simulink library "inp"  (R2021b)
settings: Solver=VariableStepAuto  StartTime=0.0  StopTime=10.0  RelTol=1e-3
undefined symbols (not defined in the file): C_TASK_5MS_S, FALSE, KINP_AcoreReadyToSlp_flg_ovrdflg, KINP_AcoreReadyToSlp_flg_ovrdval, KINP_AllowMovThd_OTA_enum_ovrdflg, KINP_AllowMovThd_OTA_enum_ovrdval, KINP_APSAngleTarget_Deg_ovrdflg, KINP_APSAngleTarget_Deg_ovrdval, KINP_APSDecReq_mps2_ovrdflg, KINP_APSDecReq_mps2_ovrdval, KINP_APSDecReqA_flg_ovrdflg, KINP_APSDecReqA_flg_ovrdval, KINP_APSDFLL_cm_ovrdflg, KINP_APSDFLL_cm_ovrdval, KINP_APSDFLR_cm_ovrdflg, KINP_APSDFLR_cm_ovrdval, KINP_APSDRLL_cm_ovrdflg, KINP_APSDRLL_cm_ovrdval, KINP_APSDRLR_cm_ovrdflg, KINP_APSDRLR_cm_ovrdval, KINP_APSExitCondition_enum_ovrdflg, KINP_APSExitCondition_enum_ovrdval, KINP_APSHWVer_enum_ovrdflg, KINP_APSHWVer_enum_ovrdval, KINP_APSProgressPCT_pct_ovrdflg, KINP_APSProgressPCT_pct_ovrdval, KINP_APSPwrReq_enum_ovrdflg, KINP_APSPwrReq_enum_ovrdval, KINP_APSReq_enum_ovrdflg, KINP_APSReq_enum_ovrdval, KINP_APSRQDisplay_enum_ovrdflg, KINP_APSRQDisplay_enum_ovrdval, KINP_APSRqEPASCtrl_flg_ovrdflg, KINP_APSRqEPASCtrl_flg_ovrdval, KINP_APSShiftPosnReq_enum_ovrdval, KINP_APSShiftPosnReq_enum_ovrflg, KINP_APSSpeedCMD_kph_ovrdval, KINP_APSSpeedCMD_kph_ovrflg, KINP_APSStaSystem_enum_ovrdflg, KINP_APSStaSystem_enum_ovrdval, KINP_APSSWVer_enum_ovrdflg, KINP_APSSWVer_enum_ovrdval, KINP_APSVMCReqA_flg_ovrdval, KINP_APSVMCReqA_flg_ovrflg, KINP_APSVRqEPASCtrl_flg_ovrdflg, KINP_APSVRqEPASCtrl_flg_ovrdval, KINP_AuxBattVolmV_mV_ovrdflg, KINP_AuxBattVolmV_mV_ovrdval, KINP_BTConnectSta_enum_ovrdflg, KINP_BTConnectSta_enum_ovrdval, KINP_CAASSta_enum_ovrdflg, KINP_CAASSta_enum_ovrdval, KINP_CAASVMCReqA_flg_ovrdval, KINP_CAASVMCReqA_flg_ovrflg, KINP_CAN1BusOff_flg_ovrdflg, KINP_CAN1BusOff_flg_ovrdval, KINP_CAN2BusOff_flg_ovrdflg, KINP_CAN2BusOff_flg_ovrdval, KINP_CAN3BusOff_flg_ovrdflg, KINP_CAN3BusOff_flg_ovrdval ... (+158)
libraries: FVT_lib x184, hcu_lib x1
(part 8 of 8)

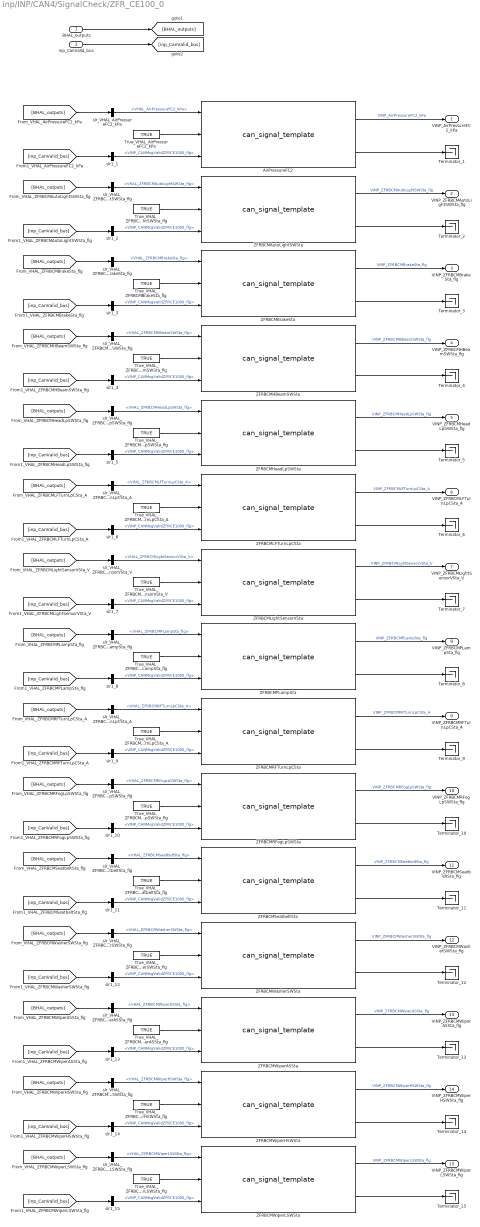
== system inp/INP/CAN4/SignalCheck/ZFR_CE100_0 ==
  BHAL_outputs : Inport
  inp_CanValid_bus : Inport  Port=2
  AirPressureFC2 : FVT_lib/inp/can_signal_template  SystemSampleTime=-1  VariantActivationTime=update diagram  Latency=0  AutoFrameSizeCalculation=off
      link override defval: Value=KINP_AirPressureFC2_kPa_defval
      link override ovrdflg: Value=KINP_AirPressureFC2_kPa_ovrdflg
      link override ovrdval: Value=KINP_AirPressureFC2_kPa_ovrdval
  Terminator_{1..15} (15 alike) : Terminator
  True_VHAL_AirPressureFC2_kPa : Constant  Value=TRUE  OutDataTypeStr=boolean
  True_VHAL_ZFRBCMAutoLightSWSta_flg : Constant  Value=TRUE  OutDataTypeStr=boolean
  True_VHAL_ZFRBCMBrakeSta_flg : Constant  Value=TRUE  OutDataTypeStr=boolean
  True_VHAL_ZFRBCMHBeamSWSta_flg : Constant  Value=TRUE  OutDataTypeStr=boolean
  True_VHAL_ZFRBCMHeadLpSWSta_flg : Constant  Value=TRUE  OutDataTypeStr=boolean
  True_VHAL_ZFRBCMLFTurnLpCSta_A : Constant  Value=TRUE  OutDataTypeStr=boolean
  True_VHAL_ZFRBCMLightSensorVSta_V : Constant  Value=TRUE  OutDataTypeStr=boolean
  True_VHAL_ZFRBCMPLampSta_flg : Constant  Value=TRUE  OutDataTypeStr=boolean
  True_VHAL_ZFRBCMRFTurnLpCSta_A : Constant  Value=TRUE  OutDataTypeStr=boolean
  True_VHAL_ZFRBCMRFogLpSWSta_flg : Constant  Value=TRUE  OutDataTypeStr=boolean
  True_VHAL_ZFRBCMSeatbeltSta_flg : Constant  Value=TRUE  OutDataTypeStr=boolean
  True_VHAL_ZFRBCMWasherSWSta_flg : Constant  Value=TRUE  OutDataTypeStr=boolean
  True_VHAL_ZFRBCMWiperASSta_flg : Constant  Value=TRUE  OutDataTypeStr=boolean
  True_VHAL_ZFRBCMWiperHSWSta_flg : Constant  Value=TRUE  OutDataTypeStr=boolean
  True_VHAL_ZFRBCMWiperLSWSta_flg : Constant  Value=TRUE  OutDataTypeStr=boolean
  ZFRBCMAutoLightSWSta : FVT_lib/inp/can_signal_template  SystemSampleTime=-1  VariantActivationTime=update diagram  Latency=0  AutoFrameSizeCalculation=off
      link override defval: Value=KINP_ZFRBCMAutoLightSWSta_flg_defval
      link override ovrdflg: Value=KINP_ZFRBCMAutoLightSWSta_flg_ovrdflg
      link override ovrdval: Value=KINP_ZFRBCMAutoLightSWSta_flg_ovrdval
  ZFRBCMBrakeSta : FVT_lib/inp/can_signal_template  SystemSampleTime=-1  VariantActivationTime=update diagram  Latency=0  AutoFrameSizeCalculation=off
      link override defval: Value=KINP_ZFRBCMBrakeSta_flg_defval
      link override ovrdflg: Value=KINP_ZFRBCMBrakeSta_flg_ovrdflg
      link override ovrdval: Value=KINP_ZFRBCMBrakeSta_flg_ovrdval
  ZFRBCMHBeamSWSta : FVT_lib/inp/can_signal_template  SystemSampleTime=-1  VariantActivationTime=update diagram  Latency=0  AutoFrameSizeCalculation=off
      link override defval: Value=KINP_ZFRBCMHBeamSWSta_flg_defval
      link override ovrdflg: Value=KINP_ZFRBCMHBeamSWSta_flg_ovrdflg
      link override ovrdval: Value=KINP_ZFRBCMHBeamSWSta_flg_ovrdval
  ZFRBCMHeadLpSWSta : FVT_lib/inp/can_signal_template  SystemSampleTime=-1  VariantActivationTime=update diagram  Latency=0  AutoFrameSizeCalculation=off
      link override defval: Value=KINP_ZFRBCMHeadLpSWSta_flg_defval
      link override ovrdflg: Value=KINP_ZFRBCMHeadLpSWSta_flg_ovrdflg
      link override ovrdval: Value=KINP_ZFRBCMHeadLpSWSta_flg_ovrdval
  ZFRBCMLFTurnLpCSta : FVT_lib/inp/can_signal_template  SystemSampleTime=-1  VariantActivationTime=update diagram  Latency=0  AutoFrameSizeCalculation=off
      link override defval: Value=KINP_ZFRBCMLFTurnLpCSta_A_defval
      link override ovrdflg: Value=KINP_ZFRBCMLFTurnLpCSta_A_ovrdflg
      link override ovrdval: Value=KINP_ZFRBCMLFTurnLpCSta_A_ovrdval
  ZFRBCMLightSensorVSta : FVT_lib/inp/can_signal_template  SystemSampleTime=-1  VariantActivationTime=update diagram  Latency=0  AutoFrameSizeCalculation=off
      link override defval: Value=KINP_ZFRBCMLightSensorVSta_V_defval
      link override ovrdflg: Value=KINP_ZFRBCMLightSensorVSta_V_ovrdflg
      link override ovrdval: Value=KINP_ZFRBCMLightSensorVSta_V_ovrdval
  ZFRBCMPLampSta : FVT_lib/inp/can_signal_template  SystemSampleTime=-1  VariantActivationTime=update diagram  Latency=0  AutoFrameSizeCalculation=off
      link override defval: Value=KINP_ZFRBCMPLampSta_flg_defval
      link override ovrdflg: Value=KINP_ZFRBCMPLampSta_flg_ovrdflg
      link override ovrdval: Value=KINP_ZFRBCMPLampSta_flg_ovrdval
  ZFRBCMRFTurnLpCSta : FVT_lib/inp/can_signal_template  SystemSampleTime=-1  VariantActivationTime=update diagram  Latency=0  AutoFrameSizeCalculation=off
      link override defval: Value=KINP_ZFRBCMRFTurnLpCSta_A_defval
      link override ovrdflg: Value=KINP_ZFRBCMRFTurnLpCSta_A_ovrdflg
      link override ovrdval: Value=KINP_ZFRBCMRFTurnLpCSta_A_ovrdval
  ZFRBCMRFogLpSWSta : FVT_lib/inp/can_signal_template  SystemSampleTime=-1  VariantActivationTime=update diagram  Latency=0  AutoFrameSizeCalculation=off
      link override defval: Value=KINP_ZFRBCMRFogLpSWSta_flg_defval
      link override ovrdflg: Value=KINP_ZFRBCMRFogLpSWSta_flg_ovrdflg
      link override ovrdval: Value=KINP_ZFRBCMRFogLpSWSta_flg_ovrdval
  ZFRBCMSeatbeltSta : FVT_lib/inp/can_signal_template  SystemSampleTime=-1  VariantActivationTime=update diagram  Latency=0  AutoFrameSizeCalculation=off
      link override defval: Value=KINP_ZFRBCMSeatbeltSta_flg_defval
      link override ovrdflg: Value=KINP_ZFRBCMSeatbeltSta_flg_ovrdflg
      link override ovrdval: Value=KINP_ZFRBCMSeatbeltSta_flg_ovrdval
  ZFRBCMWasherSWSta : FVT_lib/inp/can_signal_template  SystemSampleTime=-1  VariantActivationTime=update diagram  Latency=0  AutoFrameSizeCalculation=off
      link override defval: Value=KINP_ZFRBCMWasherSWSta_flg_defval
      link override ovrdflg: Value=KINP_ZFRBCMWasherSWSta_flg_ovrdflg
      link override ovrdval: Value=KINP_ZFRBCMWasherSWSta_flg_ovrdval
  ZFRBCMWiperASSta : FVT_lib/inp/can_signal_template  SystemSampleTime=-1  VariantActivationTime=update diagram  Latency=0  AutoFrameSizeCalculation=off
      link override defval: Value=KINP_ZFRBCMWiperASSta_flg_defval
      link override ovrdflg: Value=KINP_ZFRBCMWiperASSta_flg_ovrdflg
      link override ovrdval: Value=KINP_ZFRBCMWiperASSta_flg_ovrdval
  ZFRBCMWiperHSWSta : FVT_lib/inp/can_signal_template  SystemSampleTime=-1  VariantActivationTime=update diagram  Latency=0  AutoFrameSizeCalculation=off
      link override defval: Value=KINP_ZFRBCMWiperHSWSta_flg_defval
      link override ovrdflg: Value=KINP_ZFRBCMWiperHSWSta_flg_ovrdflg
      link override ovrdval: Value=KINP_ZFRBCMWiperHSWSta_flg_ovrdval
  ZFRBCMWiperLSWSta : FVT_lib/inp/can_signal_template  SystemSampleTime=-1  VariantActivationTime=update diagram  Latency=0  AutoFrameSizeCalculation=off
      link override defval: Value=KINP_ZFRBCMWiperLSWSta_flg_defval
      link override ovrdflg: Value=KINP_ZFRBCMWiperLSWSta_flg_ovrdflg
      link override ovrdval: Value=KINP_ZFRBCMWiperLSWSta_flg_ovrdval
  slr1_{1..15} (15 alike) : BusSelector  OutputSignals=VINP_CANMsgValidZFRCE1000_flg
  slr_VHAL_AirPressureFC2_kPa : BusSelector  OutputSignals=VHAL_AirPressureFC2_kPa
  slr_VHAL_ZFRBCMAutoLightSWSta_flg : BusSelector  OutputSignals=VHAL_ZFRBCMAutoLightSWSta_flg
  slr_VHAL_ZFRBCMBrakeSta_flg : BusSelector  OutputSignals=VHAL_ZFRBCMBrakeSta_flg
  slr_VHAL_ZFRBCMHBeamSWSta_flg : BusSelector  OutputSignals=VHAL_ZFRBCMHBeamSWSta_flg
  slr_VHAL_ZFRBCMHeadLpSWSta_flg : BusSelector  OutputSignals=VHAL_ZFRBCMHeadLpSWSta_flg
  slr_VHAL_ZFRBCMLFTurnLpCSta_A : BusSelector  OutputSignals=VHAL_ZFRBCMLFTurnLpCSta_A
  slr_VHAL_ZFRBCMLightSensorVSta_V : BusSelector  OutputSignals=VHAL_ZFRBCMLightSensorVSta_V
  slr_VHAL_ZFRBCMPLampSta_flg : BusSelector  OutputSignals=VHAL_ZFRBCMPLampSta_flg
  slr_VHAL_ZFRBCMRFTurnLpCSta_A : BusSelector  OutputSignals=VHAL_ZFRBCMRFTurnLpCSta_A
  slr_VHAL_ZFRBCMRFogLpSWSta_flg : BusSelector  OutputSignals=VHAL_ZFRBCMRFogLpSWSta_flg
  slr_VHAL_ZFRBCMSeatbeltSta_flg : BusSelector  OutputSignals=VHAL_ZFRBCMSeatbeltSta_flg
  slr_VHAL_ZFRBCMWasherSWSta_flg : BusSelector  OutputSignals=VHAL_ZFRBCMWasherSWSta_flg
  slr_VHAL_ZFRBCMWiperASSta_flg : BusSelector  OutputSignals=VHAL_ZFRBCMWiperASSta_flg
  slr_VHAL_ZFRBCMWiperHSWSta_flg : BusSelector  OutputSignals=VHAL_ZFRBCMWiperHSWSta_flg
  slr_VHAL_ZFRBCMWiperLSWSta_flg : BusSelector  OutputSignals=VHAL_ZFRBCMWiperLSWSta_flg
  VINP_AirPressureFC2_kPa : Outport
  VINP_ZFRBCMAutoLightSWSta_flg : Outport  Port=2
  VINP_ZFRBCMBrakeSta_flg : Outport  Port=3
  VINP_ZFRBCMHBeamSWSta_flg : Outport  Port=4
  VINP_ZFRBCMHeadLpSWSta_flg : Outport  Port=5
  VINP_ZFRBCMLFTurnLpCSta_A : Outport  Port=6
  VINP_ZFRBCMLightSensorVSta_V : Outport  Port=7
  VINP_ZFRBCMPLampSta_flg : Outport  Port=8
  VINP_ZFRBCMRFTurnLpCSta_A : Outport  Port=9
  VINP_ZFRBCMRFogLpSWSta_flg : Outport  Port=10
  VINP_ZFRBCMSeatbeltSta_flg : Outport  Port=11
  VINP_ZFRBCMWasherSWSta_flg : Outport  Port=12
  VINP_ZFRBCMWiperASSta_flg : Outport  Port=13
  VINP_ZFRBCMWiperHSWSta_flg : Outport  Port=14
  VINP_ZFRBCMWiperLSWSta_flg : Outport  Port=15
  wires:
  BHAL_outputs/1 -> [BHAL_outputs]
  inp_CanValid_bus/1 -> [inp_CanValid_bus]
  [BHAL_outputs] -> slr_VHAL_AirPressureFC2_kPa/1
  slr_VHAL_AirPressureFC2_kPa/1 -> AirPressureFC2/1  "<VHAL_AirPressureFC2_kPa>"
  True_VHAL_AirPressureFC2_kPa/1 -> AirPressureFC2/2
  [inp_CanValid_bus] -> slr1_1/1
  slr1_1/1 -> AirPressureFC2/3  "<VINP_CANMsgValidZFRCE1000_flg>"
  AirPressureFC2/1 -> VINP_AirPressureFC2_kPa/1  "VINP_AirPressureFC2_kPa"
  AirPressureFC2/2 -> Terminator_1/1
  [BHAL_outputs] -> slr_VHAL_ZFRBCMAutoLightSWSta_flg/1
  slr_VHAL_ZFRBCMAutoLightSWSta_flg/1 -> ZFRBCMAutoLightSWSta/1  "<VHAL_ZFRBCMAutoLightSWSta_flg>"
  True_VHAL_ZFRBCMAutoLightSWSta_flg/1 -> ZFRBCMAutoLightSWSta/2
  [inp_CanValid_bus] -> slr1_2/1
  slr1_2/1 -> ZFRBCMAutoLightSWSta/3  "<VINP_CANMsgValidZFRCE1000_flg>"
  ZFRBCMAutoLightSWSta/1 -> VINP_ZFRBCMAutoLightSWSta_flg/1  "VINP_ZFRBCMAutoLightSWSta_flg"
  ZFRBCMAutoLightSWSta/2 -> Terminator_2/1
  [BHAL_outputs] -> slr_VHAL_ZFRBCMBrakeSta_flg/1
  slr_VHAL_ZFRBCMBrakeSta_flg/1 -> ZFRBCMBrakeSta/1  "<VHAL_ZFRBCMBrakeSta_flg>"
  True_VHAL_ZFRBCMBrakeSta_flg/1 -> ZFRBCMBrakeSta/2
  [inp_CanValid_bus] -> slr1_3/1
  slr1_3/1 -> ZFRBCMBrakeSta/3  "<VINP_CANMsgValidZFRCE1000_flg>"
  ZFRBCMBrakeSta/1 -> VINP_ZFRBCMBrakeSta_flg/1  "VINP_ZFRBCMBrakeSta_flg"
  ZFRBCMBrakeSta/2 -> Terminator_3/1
  [BHAL_outputs] -> slr_VHAL_ZFRBCMHBeamSWSta_flg/1
  slr_VHAL_ZFRBCMHBeamSWSta_flg/1 -> ZFRBCMHBeamSWSta/1  "<VHAL_ZFRBCMHBeamSWSta_flg>"
  True_VHAL_ZFRBCMHBeamSWSta_flg/1 -> ZFRBCMHBeamSWSta/2
  [inp_CanValid_bus] -> slr1_4/1
  slr1_4/1 -> ZFRBCMHBeamSWSta/3  "<VINP_CANMsgValidZFRCE1000_flg>"
  ZFRBCMHBeamSWSta/1 -> VINP_ZFRBCMHBeamSWSta_flg/1  "VINP_ZFRBCMHBeamSWSta_flg"
  ZFRBCMHBeamSWSta/2 -> Terminator_4/1
  [BHAL_outputs] -> slr_VHAL_ZFRBCMHeadLpSWSta_flg/1
  slr_VHAL_ZFRBCMHeadLpSWSta_flg/1 -> ZFRBCMHeadLpSWSta/1  "<VHAL_ZFRBCMHeadLpSWSta_flg>"
  True_VHAL_ZFRBCMHeadLpSWSta_flg/1 -> ZFRBCMHeadLpSWSta/2
  [inp_CanValid_bus] -> slr1_5/1
  slr1_5/1 -> ZFRBCMHeadLpSWSta/3  "<VINP_CANMsgValidZFRCE1000_flg>"
  ZFRBCMHeadLpSWSta/1 -> VINP_ZFRBCMHeadLpSWSta_flg/1  "VINP_ZFRBCMHeadLpSWSta_flg"
  ZFRBCMHeadLpSWSta/2 -> Terminator_5/1
  [BHAL_outputs] -> slr_VHAL_ZFRBCMLFTurnLpCSta_A/1
  slr_VHAL_ZFRBCMLFTurnLpCSta_A/1 -> ZFRBCMLFTurnLpCSta/1  "<VHAL_ZFRBCMLFTurnLpCSta_A>"
  True_VHAL_ZFRBCMLFTurnLpCSta_A/1 -> ZFRBCMLFTurnLpCSta/2
  [inp_CanValid_bus] -> slr1_6/1
  slr1_6/1 -> ZFRBCMLFTurnLpCSta/3  "<VINP_CANMsgValidZFRCE1000_flg>"
  ZFRBCMLFTurnLpCSta/1 -> VINP_ZFRBCMLFTurnLpCSta_A/1  "VINP_ZFRBCMLFTurnLpCSta_A"
  ZFRBCMLFTurnLpCSta/2 -> Terminator_6/1
  [BHAL_outputs] -> slr_VHAL_ZFRBCMLightSensorVSta_V/1
  slr_VHAL_ZFRBCMLightSensorVSta_V/1 -> ZFRBCMLightSensorVSta/1  "<VHAL_ZFRBCMLightSensorVSta_V>"
  True_VHAL_ZFRBCMLightSensorVSta_V/1 -> ZFRBCMLightSensorVSta/2
  [inp_CanValid_bus] -> slr1_7/1
  slr1_7/1 -> ZFRBCMLightSensorVSta/3  "<VINP_CANMsgValidZFRCE1000_flg>"
  ZFRBCMLightSensorVSta/1 -> VINP_ZFRBCMLightSensorVSta_V/1  "VINP_ZFRBCMLightSensorVSta_V"
  ZFRBCMLightSensorVSta/2 -> Terminator_7/1
  [BHAL_outputs] -> slr_VHAL_ZFRBCMPLampSta_flg/1
  slr_VHAL_ZFRBCMPLampSta_flg/1 -> ZFRBCMPLampSta/1  "<VHAL_ZFRBCMPLampSta_flg>"
  True_VHAL_ZFRBCMPLampSta_flg/1 -> ZFRBCMPLampSta/2
  [inp_CanValid_bus] -> slr1_8/1
  slr1_8/1 -> ZFRBCMPLampSta/3  "<VINP_CANMsgValidZFRCE1000_flg>"
  ZFRBCMPLampSta/1 -> VINP_ZFRBCMPLampSta_flg/1  "VINP_ZFRBCMPLampSta_flg"
  ZFRBCMPLampSta/2 -> Terminator_8/1
  [BHAL_outputs] -> slr_VHAL_ZFRBCMRFTurnLpCSta_A/1
  slr_VHAL_ZFRBCMRFTurnLpCSta_A/1 -> ZFRBCMRFTurnLpCSta/1  "<VHAL_ZFRBCMRFTurnLpCSta_A>"
  True_VHAL_ZFRBCMRFTurnLpCSta_A/1 -> ZFRBCMRFTurnLpCSta/2
  [inp_CanValid_bus] -> slr1_9/1
  slr1_9/1 -> ZFRBCMRFTurnLpCSta/3  "<VINP_CANMsgValidZFRCE1000_flg>"
  ZFRBCMRFTurnLpCSta/1 -> VINP_ZFRBCMRFTurnLpCSta_A/1  "VINP_ZFRBCMRFTurnLpCSta_A"
  ZFRBCMRFTurnLpCSta/2 -> Terminator_9/1
  [BHAL_outputs] -> slr_VHAL_ZFRBCMRFogLpSWSta_flg/1
  slr_VHAL_ZFRBCMRFogLpSWSta_flg/1 -> ZFRBCMRFogLpSWSta/1  "<VHAL_ZFRBCMRFogLpSWSta_flg>"
  True_VHAL_ZFRBCMRFogLpSWSta_flg/1 -> ZFRBCMRFogLpSWSta/2
  [inp_CanValid_bus] -> slr1_10/1
  slr1_10/1 -> ZFRBCMRFogLpSWSta/3  "<VINP_CANMsgValidZFRCE1000_flg>"
  ZFRBCMRFogLpSWSta/1 -> VINP_ZFRBCMRFogLpSWSta_flg/1  "VINP_ZFRBCMRFogLpSWSta_flg"
  ZFRBCMRFogLpSWSta/2 -> Terminator_10/1
  [BHAL_outputs] -> slr_VHAL_ZFRBCMSeatbeltSta_flg/1
  slr_VHAL_ZFRBCMSeatbeltSta_flg/1 -> ZFRBCMSeatbeltSta/1  "<VHAL_ZFRBCMSeatbeltSta_flg>"
  True_VHAL_ZFRBCMSeatbeltSta_flg/1 -> ZFRBCMSeatbeltSta/2
  [inp_CanValid_bus] -> slr1_11/1
  slr1_11/1 -> ZFRBCMSeatbeltSta/3  "<VINP_CANMsgValidZFRCE1000_flg>"
  ZFRBCMSeatbeltSta/1 -> VINP_ZFRBCMSeatbeltSta_flg/1  "VINP_ZFRBCMSeatbeltSta_flg"
  ZFRBCMSeatbeltSta/2 -> Terminator_11/1
  [BHAL_outputs] -> slr_VHAL_ZFRBCMWasherSWSta_flg/1
  slr_VHAL_ZFRBCMWasherSWSta_flg/1 -> ZFRBCMWasherSWSta/1  "<VHAL_ZFRBCMWasherSWSta_flg>"
  True_VHAL_ZFRBCMWasherSWSta_flg/1 -> ZFRBCMWasherSWSta/2
  [inp_CanValid_bus] -> slr1_12/1
  slr1_12/1 -> ZFRBCMWasherSWSta/3  "<VINP_CANMsgValidZFRCE1000_flg>"
  ZFRBCMWasherSWSta/1 -> VINP_ZFRBCMWasherSWSta_flg/1  "VINP_ZFRBCMWasherSWSta_flg"
  ZFRBCMWasherSWSta/2 -> Terminator_12/1
  [BHAL_outputs] -> slr_VHAL_ZFRBCMWiperASSta_flg/1
  slr_VHAL_ZFRBCMWiperASSta_flg/1 -> ZFRBCMWiperASSta/1  "<VHAL_ZFRBCMWiperASSta_flg>"
  True_VHAL_ZFRBCMWiperASSta_flg/1 -> ZFRBCMWiperASSta/2
  [inp_CanValid_bus] -> slr1_13/1
  slr1_13/1 -> ZFRBCMWiperASSta/3  "<VINP_CANMsgValidZFRCE1000_flg>"
  ZFRBCMWiperASSta/1 -> VINP_ZFRBCMWiperASSta_flg/1  "VINP_ZFRBCMWiperASSta_flg"
  ZFRBCMWiperASSta/2 -> Terminator_13/1
  [BHAL_outputs] -> slr_VHAL_ZFRBCMWiperHSWSta_flg/1
  slr_VHAL_ZFRBCMWiperHSWSta_flg/1 -> ZFRBCMWiperHSWSta/1  "<VHAL_ZFRBCMWiperHSWSta_flg>"
  True_VHAL_ZFRBCMWiperHSWSta_flg/1 -> ZFRBCMWiperHSWSta/2
  [inp_CanValid_bus] -> slr1_14/1
  slr1_14/1 -> ZFRBCMWiperHSWSta/3  "<VINP_CANMsgValidZFRCE1000_flg>"
  ZFRBCMWiperHSWSta/1 -> VINP_ZFRBCMWiperHSWSta_flg/1  "VINP_ZFRBCMWiperHSWSta_flg"
  ZFRBCMWiperHSWSta/2 -> Terminator_14/1
  [BHAL_outputs] -> slr_VHAL_ZFRBCMWiperLSWSta_flg/1
  slr_VHAL_ZFRBCMWiperLSWSta_flg/1 -> ZFRBCMWiperLSWSta/1  "<VHAL_ZFRBCMWiperLSWSta_flg>"
  True_VHAL_ZFRBCMWiperLSWSta_flg/1 -> ZFRBCMWiperLSWSta/2
  [inp_CanValid_bus] -> slr1_15/1
  slr1_15/1 -> ZFRBCMWiperLSWSta/3  "<VINP_CANMsgValidZFRCE1000_flg>"
  ZFRBCMWiperLSWSta/1 -> VINP_ZFRBCMWiperLSWSta_flg/1  "VINP_ZFRBCMWiperLSWSta_flg"
  ZFRBCMWiperLSWSta/2 -> Terminator_15/1

== system inp/INP/CAN4/SignalCheck/ZRR_CE100_0 ==
  BHAL_outputs : Inport
  inp_CanValid_bus : Inport  Port=2
  Terminator_1 : Terminator
  True_VHAL_ZRRBCMAllDoorSta_enum : Constant  Value=TRUE  OutDataTypeStr=boolean
  ZRRBCMAllDoorSta : FVT_lib/inp/can_signal_template  SystemSampleTime=-1  VariantActivationTime=update diagram  Latency=0  AutoFrameSizeCalculation=off
      link override defval: Value=KINP_ZRRBCMAllDoorSta_enum_defval
      link override ovrdflg: Value=KINP_ZRRBCMAllDoorSta_enum_ovrdflg
      link override ovrdval: Value=KINP_ZRRBCMAllDoorSta_enum_ovrdval
  slr1_1 : BusSelector  OutputSignals=VINP_CANMsgValidZRRCE1000_flg
  slr_VHAL_ZRRBCMAllDoorSta_enum : BusSelector  OutputSignals=VHAL_ZRRBCMAllDoorSta_enum
  VINP_ZRRBCMAllDoorSta_enum : Outport
  wires:
  BHAL_outputs/1 -> [BHAL_outputs]
  inp_CanValid_bus/1 -> [inp_CanValid_bus]
  [BHAL_outputs] -> slr_VHAL_ZRRBCMAllDoorSta_enum/1
  slr_VHAL_ZRRBCMAllDoorSta_enum/1 -> ZRRBCMAllDoorSta/1  "<VHAL_ZRRBCMAllDoorSta_enum>"
  True_VHAL_ZRRBCMAllDoorSta_enum/1 -> ZRRBCMAllDoorSta/2
  [inp_CanValid_bus] -> slr1_1/1
  slr1_1/1 -> ZRRBCMAllDoorSta/3  "<VINP_CANMsgValidZRRCE1000_flg>"
  ZRRBCMAllDoorSta/1 -> VINP_ZRRBCMAllDoorSta_enum/1  "VINP_ZRRBCMAllDoorSta_enum"
  ZRRBCMAllDoorSta/2 -> Terminator_1/1

== system inp/INP/CAN4/SignalCheck/ZRR_CE100_1 ==
  BHAL_outputs : Inport
  inp_CanValid_bus : Inport  Port=2
  AirPressurePC3 : FVT_lib/inp/can_signal_template  SystemSampleTime=-1  VariantActivationTime=update diagram  Latency=0  AutoFrameSizeCalculation=off
      link override defval: Value=KINP_AirPressurePC3_kPa_defval
      link override ovrdflg: Value=KINP_AirPressurePC3_kPa_ovrdflg
      link override ovrdval: Value=KINP_AirPressurePC3_kPa_ovrdval
  AirPressureRC1 : FVT_lib/inp/can_signal_template  SystemSampleTime=-1  VariantActivationTime=update diagram  Latency=0  AutoFrameSizeCalculation=off
      link override defval: Value=KINP_AirPressureRC1_kPa_defval
      link override ovrdflg: Value=KINP_AirPressureRC1_kPa_ovrdflg
      link override ovrdval: Value=KINP_AirPressureRC1_kPa_ovrdval
  FDCCHASSISVCUEACPressSta : FVT_lib/inp/can_signal_template  SystemSampleTime=-1  VariantActivationTime=update diagram  Latency=0  AutoFrameSizeCalculation=off
      link override defval: Value=KINP_FDCCHASSISVCUEACPressSta_flg_defval
      link override ovrdflg: Value=KINP_FDCCHASSISVCUEACPressSta_flg_ovrdflg
      link override ovrdval: Value=KINP_FDCCHASSISVCUEACPressSta_flg_ovrdval
  Terminator_{1..9} (9 alike) : Terminator
  True_VHAL_AirPressurePC3_kPa : Constant  Value=TRUE  OutDataTypeStr=boolean
  True_VHAL_AirPressureRC1_kPa : Constant  Value=TRUE  OutDataTypeStr=boolean
  True_VHAL_FDCCHASSISVCUEACPressSta_flg : Constant  Value=TRUE  OutDataTypeStr=boolean
  True_VHAL_ZRRBCMCallingSWSta_flg : Constant  Value=TRUE  OutDataTypeStr=boolean
  True_VHAL_ZRRBCMLRTurnLpCSta_A : Constant  Value=TRUE  OutDataTypeStr=boolean
  True_VHAL_ZRRBCMPLampSta_flg : Constant  Value=TRUE  OutDataTypeStr=boolean
  True_VHAL_ZRRBCMRRTurnLpCSta_A : Constant  Value=TRUE  OutDataTypeStr=boolean
  True_VHAL_ZRRBCMSTOPSW2Sta_flg : Constant  Value=TRUE  OutDataTypeStr=boolean
  True_VHAL_ZRRBCMSTOPSWSta_flg : Constant  Value=TRUE  OutDataTypeStr=boolean
  ZRRBCMCallingSWSta : FVT_lib/inp/can_signal_template  SystemSampleTime=-1  VariantActivationTime=update diagram  Latency=0  AutoFrameSizeCalculation=off
      link override defval: Value=KINP_ZRRBCMCallingSWSta_flg_defval
      link override ovrdflg: Value=KINP_ZRRBCMCallingSWSta_flg_ovrdflg
      link override ovrdval: Value=KINP_ZRRBCMCallingSWSta_flg_ovrdval
  ZRRBCMLRTurnLpCSta : FVT_lib/inp/can_signal_template  SystemSampleTime=-1  VariantActivationTime=update diagram  Latency=0  AutoFrameSizeCalculation=off
      link override defval: Value=KINP_ZRRBCMLRTurnLpCSta_A_defval
      link override ovrdflg: Value=KINP_ZRRBCMLRTurnLpCSta_A_ovrdflg
      link override ovrdval: Value=KINP_ZRRBCMLRTurnLpCSta_A_ovrdval
  ZRRBCMPLampSta : FVT_lib/inp/can_signal_template  SystemSampleTime=-1  VariantActivationTime=update diagram  Latency=0  AutoFrameSizeCalculation=off
      link override defval: Value=KINP_ZRRBCMPLampSta_flg_defval
      link override ovrdflg: Value=KINP_ZRRBCMPLampSta_flg_ovrdflg
      link override ovrdval: Value=KINP_ZRRBCMPLampSta_flg_ovrdval
  ZRRBCMRRTurnLpCSta : FVT_lib/inp/can_signal_template  SystemSampleTime=-1  VariantActivationTime=update diagram  Latency=0  AutoFrameSizeCalculation=off
      link override defval: Value=KINP_ZRRBCMRRTurnLpCSta_A_defval
      link override ovrdflg: Value=KINP_ZRRBCMRRTurnLpCSta_A_ovrdflg
      link override ovrdval: Value=KINP_ZRRBCMRRTurnLpCSta_A_ovrdval
  ZRRBCMSTOPSW2Sta : FVT_lib/inp/can_signal_template  SystemSampleTime=-1  VariantActivationTime=update diagram  Latency=0  AutoFrameSizeCalculation=off
      link override defval: Value=KINP_ZRRBCMSTOPSW2Sta_flg_defval
      link override ovrdflg: Value=KINP_ZRRBCMSTOPSW2Sta_flg_ovrdflg
      link override ovrdval: Value=KINP_ZRRBCMSTOPSW2Sta_flg_ovrdval
  ZRRBCMSTOPSWSta : FVT_lib/inp/can_signal_template  SystemSampleTime=-1  VariantActivationTime=update diagram  Latency=0  AutoFrameSizeCalculation=off
      link override defval: Value=KINP_ZRRBCMSTOPSWSta_flg_defval
      link override ovrdflg: Value=KINP_ZRRBCMSTOPSWSta_flg_ovrdflg
      link override ovrdval: Value=KINP_ZRRBCMSTOPSWSta_flg_ovrdval
  slr1_{1..9} (9 alike) : BusSelector  OutputSignals=VINP_CANMsgValidZRRCE1001_flg
  slr_VHAL_AirPressurePC3_kPa : BusSelector  OutputSignals=VHAL_AirPressurePC3_kPa
  slr_VHAL_AirPressureRC1_kPa : BusSelector  OutputSignals=VHAL_AirPressureRC1_kPa
  slr_VHAL_FDCCHASSISVCUEACPressSta_flg : BusSelector  OutputSignals=VHAL_FDCCHASSISVCUEACPressSta_flg
  slr_VHAL_ZRRBCMCallingSWSta_flg : BusSelector  OutputSignals=VHAL_ZRRBCMCallingSWSta_flg
  slr_VHAL_ZRRBCMLRTurnLpCSta_A : BusSelector  OutputSignals=VHAL_ZRRBCMLRTurnLpCSta_A
  slr_VHAL_ZRRBCMPLampSta_flg : BusSelector  OutputSignals=VHAL_ZRRBCMPLampSta_flg
  slr_VHAL_ZRRBCMRRTurnLpCSta_A : BusSelector  OutputSignals=VHAL_ZRRBCMRRTurnLpCSta_A
  slr_VHAL_ZRRBCMSTOPSW2Sta_flg : BusSelector  OutputSignals=VHAL_ZRRBCMSTOPSW2Sta_flg
  slr_VHAL_ZRRBCMSTOPSWSta_flg : BusSelector  OutputSignals=VHAL_ZRRBCMSTOPSWSta_flg
  VINP_AirPressurePC3_kPa : Outport
  VINP_AirPressureRC1_kPa : Outport  Port=2
  VINP_FDCCHASSISVCUEACPressSta_flg : Outport  Port=3
  VINP_ZRRBCMCallingSWSta_flg : Outport  Port=4
  VINP_ZRRBCMLRTurnLpCSta_A : Outport  Port=5
  VINP_ZRRBCMPLampSta_flg : Outport  Port=6
  VINP_ZRRBCMRRTurnLpCSta_A : Outport  Port=7
  VINP_ZRRBCMSTOPSW2Sta_flg : Outport  Port=8
  VINP_ZRRBCMSTOPSWSta_flg : Outport  Port=9
  wires:
  BHAL_outputs/1 -> [BHAL_outputs]
  inp_CanValid_bus/1 -> [inp_CanValid_bus]
  [BHAL_outputs] -> slr_VHAL_AirPressurePC3_kPa/1
  slr_VHAL_AirPressurePC3_kPa/1 -> AirPressurePC3/1  "<VHAL_AirPressurePC3_kPa>"
  True_VHAL_AirPressurePC3_kPa/1 -> AirPressurePC3/2
  [inp_CanValid_bus] -> slr1_1/1
  slr1_1/1 -> AirPressurePC3/3  "<VINP_CANMsgValidZRRCE1001_flg>"
  AirPressurePC3/1 -> VINP_AirPressurePC3_kPa/1  "VINP_AirPressurePC3_kPa"
  AirPressurePC3/2 -> Terminator_1/1
  [BHAL_outputs] -> slr_VHAL_AirPressureRC1_kPa/1
  slr_VHAL_AirPressureRC1_kPa/1 -> AirPressureRC1/1  "<VHAL_AirPressureRC1_kPa>"
  True_VHAL_AirPressureRC1_kPa/1 -> AirPressureRC1/2
  [inp_CanValid_bus] -> slr1_2/1
  slr1_2/1 -> AirPressureRC1/3  "<VINP_CANMsgValidZRRCE1001_flg>"
  AirPressureRC1/1 -> VINP_AirPressureRC1_kPa/1  "VINP_AirPressureRC1_kPa"
  AirPressureRC1/2 -> Terminator_2/1
  [BHAL_outputs] -> slr_VHAL_FDCCHASSISVCUEACPressSta_flg/1
  slr_VHAL_FDCCHASSISVCUEACPressSta_flg/1 -> FDCCHASSISVCUEACPressSta/1  "<VHAL_FDCCHASSISVCUEACPressSta_flg>"
  True_VHAL_FDCCHASSISVCUEACPressSta_flg/1 -> FDCCHASSISVCUEACPressSta/2
  [inp_CanValid_bus] -> slr1_3/1
  slr1_3/1 -> FDCCHASSISVCUEACPressSta/3  "<VINP_CANMsgValidZRRCE1001_flg>"
  FDCCHASSISVCUEACPressSta/1 -> VINP_FDCCHASSISVCUEACPressSta_flg/1  "VINP_FDCCHASSISVCUEACPressSta_flg"
  FDCCHASSISVCUEACPressSta/2 -> Terminator_3/1
  [BHAL_outputs] -> slr_VHAL_ZRRBCMCallingSWSta_flg/1
  slr_VHAL_ZRRBCMCallingSWSta_flg/1 -> ZRRBCMCallingSWSta/1  "<VHAL_ZRRBCMCallingSWSta_flg>"
  True_VHAL_ZRRBCMCallingSWSta_flg/1 -> ZRRBCMCallingSWSta/2
  [inp_CanValid_bus] -> slr1_4/1
  slr1_4/1 -> ZRRBCMCallingSWSta/3  "<VINP_CANMsgValidZRRCE1001_flg>"
  ZRRBCMCallingSWSta/1 -> VINP_ZRRBCMCallingSWSta_flg/1  "VINP_ZRRBCMCallingSWSta_flg"
  ZRRBCMCallingSWSta/2 -> Terminator_4/1
  [BHAL_outputs] -> slr_VHAL_ZRRBCMLRTurnLpCSta_A/1
  slr_VHAL_ZRRBCMLRTurnLpCSta_A/1 -> ZRRBCMLRTurnLpCSta/1  "<VHAL_ZRRBCMLRTurnLpCSta_A>"
  True_VHAL_ZRRBCMLRTurnLpCSta_A/1 -> ZRRBCMLRTurnLpCSta/2
  [inp_CanValid_bus] -> slr1_5/1
  slr1_5/1 -> ZRRBCMLRTurnLpCSta/3  "<VINP_CANMsgValidZRRCE1001_flg>"
  ZRRBCMLRTurnLpCSta/1 -> VINP_ZRRBCMLRTurnLpCSta_A/1  "VINP_ZRRBCMLRTurnLpCSta_A"
  ZRRBCMLRTurnLpCSta/2 -> Terminator_5/1
  [BHAL_outputs] -> slr_VHAL_ZRRBCMPLampSta_flg/1
  slr_VHAL_ZRRBCMPLampSta_flg/1 -> ZRRBCMPLampSta/1  "<VHAL_ZRRBCMPLampSta_flg>"
  True_VHAL_ZRRBCMPLampSta_flg/1 -> ZRRBCMPLampSta/2
  [inp_CanValid_bus] -> slr1_6/1
  slr1_6/1 -> ZRRBCMPLampSta/3  "<VINP_CANMsgValidZRRCE1001_flg>"
  ZRRBCMPLampSta/1 -> VINP_ZRRBCMPLampSta_flg/1  "VINP_ZRRBCMPLampSta_flg"
  ZRRBCMPLampSta/2 -> Terminator_6/1
  [BHAL_outputs] -> slr_VHAL_ZRRBCMRRTurnLpCSta_A/1
  slr_VHAL_ZRRBCMRRTurnLpCSta_A/1 -> ZRRBCMRRTurnLpCSta/1  "<VHAL_ZRRBCMRRTurnLpCSta_A>"
  True_VHAL_ZRRBCMRRTurnLpCSta_A/1 -> ZRRBCMRRTurnLpCSta/2
  [inp_CanValid_bus] -> slr1_7/1
  slr1_7/1 -> ZRRBCMRRTurnLpCSta/3  "<VINP_CANMsgValidZRRCE1001_flg>"
  ZRRBCMRRTurnLpCSta/1 -> VINP_ZRRBCMRRTurnLpCSta_A/1  "VINP_ZRRBCMRRTurnLpCSta_A"
  ZRRBCMRRTurnLpCSta/2 -> Terminator_7/1
  [BHAL_outputs] -> slr_VHAL_ZRRBCMSTOPSW2Sta_flg/1
  slr_VHAL_ZRRBCMSTOPSW2Sta_flg/1 -> ZRRBCMSTOPSW2Sta/1  "<VHAL_ZRRBCMSTOPSW2Sta_flg>"
  True_VHAL_ZRRBCMSTOPSW2Sta_flg/1 -> ZRRBCMSTOPSW2Sta/2
  [inp_CanValid_bus] -> slr1_8/1
  slr1_8/1 -> ZRRBCMSTOPSW2Sta/3  "<VINP_CANMsgValidZRRCE1001_flg>"
  ZRRBCMSTOPSW2Sta/1 -> VINP_ZRRBCMSTOPSW2Sta_flg/1  "VINP_ZRRBCMSTOPSW2Sta_flg"
  ZRRBCMSTOPSW2Sta/2 -> Terminator_8/1
  [BHAL_outputs] -> slr_VHAL_ZRRBCMSTOPSWSta_flg/1
  slr_VHAL_ZRRBCMSTOPSWSta_flg/1 -> ZRRBCMSTOPSWSta/1  "<VHAL_ZRRBCMSTOPSWSta_flg>"
  True_VHAL_ZRRBCMSTOPSWSta_flg/1 -> ZRRBCMSTOPSWSta/2
  [inp_CanValid_bus] -> slr1_9/1
  slr1_9/1 -> ZRRBCMSTOPSWSta/3  "<VINP_CANMsgValidZRRCE1001_flg>"
  ZRRBCMSTOPSWSta/1 -> VINP_ZRRBCMSTOPSWSta_flg/1  "VINP_ZRRBCMSTOPSWSta_flg"
  ZRRBCMSTOPSWSta/2 -> Terminator_9/1

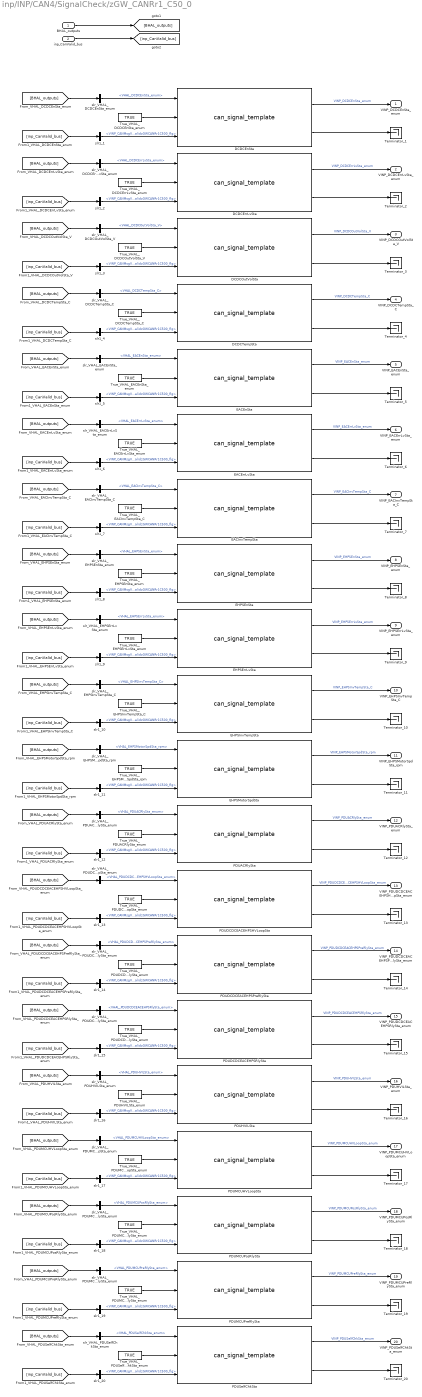
== system inp/INP/CAN4/SignalCheck/zGW_CANRr1_C50_0 ==
  BHAL_outputs : Inport
  inp_CanValid_bus : Inport  Port=2
  DCDCEnSta : FVT_lib/inp/can_signal_template  SystemSampleTime=-1  VariantActivationTime=update diagram  Latency=0  AutoFrameSizeCalculation=off
      link override defval: Value=KINP_DCDCEnSta_enum_defval
      link override ovrdflg: Value=KINP_DCDCEnSta_enum_ovrdflg
      link override ovrdval: Value=KINP_DCDCEnSta_enum_ovrdval
  DCDCErrLvSta : FVT_lib/inp/can_signal_template  SystemSampleTime=-1  VariantActivationTime=update diagram  Latency=0  AutoFrameSizeCalculation=off
      link override defval: Value=KINP_DCDCErrLvSta_enum_defval
      link override ovrdflg: Value=KINP_DCDCErrLvSta_enum_ovrdflg
      link override ovrdval: Value=KINP_DCDCErrLvSta_enum_ovrdval
  DCDCOutVolSta : FVT_lib/inp/can_signal_template  SystemSampleTime=-1  VariantActivationTime=update diagram  Latency=0  AutoFrameSizeCalculation=off
      link override defval: Value=KINP_DCDCOutVolSta_V_defval
      link override ovrdflg: Value=KINP_DCDCOutVolSta_V_ovrdflg
      link override ovrdval: Value=KINP_DCDCOutVolSta_V_ovrdval
  DCDCTempSta : FVT_lib/inp/can_signal_template  SystemSampleTime=-1  VariantActivationTime=update diagram  Latency=0  AutoFrameSizeCalculation=off
      link override defval: Value=KINP_DCDCTempSta_C_defval
      link override ovrdflg: Value=KINP_DCDCTempSta_C_ovrdflg
      link override ovrdval: Value=KINP_DCDCTempSta_C_ovrdval
  EACEnSta : FVT_lib/inp/can_signal_template  SystemSampleTime=-1  VariantActivationTime=update diagram  Latency=0  AutoFrameSizeCalculation=off
      link override defval: Value=KINP_EACEnSta_enum_defval
      link override ovrdflg: Value=KINP_EACEnSta_enum_ovrdflg
      link override ovrdval: Value=KINP_EACEnSta_enum_ovrdval
  EACErrLvSta : FVT_lib/inp/can_signal_template  SystemSampleTime=-1  VariantActivationTime=update diagram  Latency=0  AutoFrameSizeCalculation=off
      link override defval: Value=KINP_EACErrLvSta_enum_defval
      link override ovrdflg: Value=KINP_EACErrLvSta_enum_ovrdflg
      link override ovrdval: Value=KINP_EACErrLvSta_enum_ovrdval
  EACInvTempSta : FVT_lib/inp/can_signal_template  SystemSampleTime=-1  VariantActivationTime=update diagram  Latency=0  AutoFrameSizeCalculation=off
      link override defval: Value=KINP_EACInvTempSta_C_defval
      link override ovrdflg: Value=KINP_EACInvTempSta_C_ovrdflg
      link override ovrdval: Value=KINP_EACInvTempSta_C_ovrdval
  EHPSEnSta : FVT_lib/inp/can_signal_template  SystemSampleTime=-1  VariantActivationTime=update diagram  Latency=0  AutoFrameSizeCalculation=off
      link override defval: Value=KINP_EHPSEnSta_enum_defval
      link override ovrdflg: Value=KINP_EHPSEnSta_enum_ovrdflg
      link override ovrdval: Value=KINP_EHPSEnSta_enum_ovrdval
  EHPSErrLvSta : FVT_lib/inp/can_signal_template  SystemSampleTime=-1  VariantActivationTime=update diagram  Latency=0  AutoFrameSizeCalculation=off
      link override defval: Value=KINP_EHPSErrLvSta_enum_defval
      link override ovrdflg: Value=KINP_EHPSErrLvSta_enum_ovrdflg
      link override ovrdval: Value=KINP_EHPSErrLvSta_enum_ovrdval
  EHPSInvTempSta : FVT_lib/inp/can_signal_template  SystemSampleTime=-1  VariantActivationTime=update diagram  Latency=0  AutoFrameSizeCalculation=off
      link override defval: Value=KINP_EHPSInvTempSta_C_defval
      link override ovrdflg: Value=KINP_EHPSInvTempSta_C_ovrdflg
      link override ovrdval: Value=KINP_EHPSInvTempSta_C_ovrdval
  EHPSMotorSpdSta : FVT_lib/inp/can_signal_template  SystemSampleTime=-1  VariantActivationTime=update diagram  Latency=0  AutoFrameSizeCalculation=off
      link override defval: Value=KINP_EHPSMotorSpdSta_rpm_defval
      link override ovrdflg: Value=KINP_EHPSMotorSpdSta_rpm_ovrdflg
      link override ovrdval: Value=KINP_EHPSMotorSpdSta_rpm_ovrdval
  PDUACRlySta : FVT_lib/inp/can_signal_template  SystemSampleTime=-1  VariantActivationTime=update diagram  Latency=0  AutoFrameSizeCalculation=off
      link override defval: Value=KINP_PDUACRlySta_enum_defval
      link override ovrdflg: Value=KINP_PDUACRlySta_enum_ovrdflg
      link override ovrdval: Value=KINP_PDUACRlySta_enum_ovrdval
  PDUDCDCEACEHPSHVLoopSta : FVT_lib/inp/can_signal_template  SystemSampleTime=-1  VariantActivationTime=update diagram  Latency=0  AutoFrameSizeCalculation=off
      link override defval: Value=KINP_PDUDCDCEACEHPSHVLoopSta_enum_defval
      link override ovrdflg: Value=KINP_PDUDCDCEACEHPSHVLoopSta_enum_ovrdflg
      link override ovrdval: Value=KINP_PDUDCDCEACEHPSHVLoopSta_enum_ovrdval
  PDUDCDCEACEHPSPreRlySta : FVT_lib/inp/can_signal_template  SystemSampleTime=-1  VariantActivationTime=update diagram  Latency=0  AutoFrameSizeCalculation=off
      link override defval: Value=KINP_PDUDCDCEACEHPSPreRlySta_enum_defval
      link override ovrdflg: Value=KINP_PDUDCDCEACEHPSPreRlySta_enum_ovrdflg
      link override ovrdval: Value=KINP_PDUDCDCEACEHPSPreRlySta_enum_ovrdval
  PDUDCDCEACEHPSRlySta : FVT_lib/inp/can_signal_template  SystemSampleTime=-1  VariantActivationTime=update diagram  Latency=0  AutoFrameSizeCalculation=off
      link override defval: Value=KINP_PDUDCDCEACEHPSRlySta_enum_defval
      link override ovrdflg: Value=KINP_PDUDCDCEACEHPSRlySta_enum_ovrdflg
      link override ovrdval: Value=KINP_PDUDCDCEACEHPSRlySta_enum_ovrdval
  PDUHVILSta : FVT_lib/inp/can_signal_template  SystemSampleTime=-1  VariantActivationTime=update diagram  Latency=0  AutoFrameSizeCalculation=off
      link override defval: Value=KINP_PDUHVILSta_enum_defval
      link override ovrdflg: Value=KINP_PDUHVILSta_enum_ovrdflg
      link override ovrdval: Value=KINP_PDUHVILSta_enum_ovrdval
  PDUMCUHVLoopSta : FVT_lib/inp/can_signal_template  SystemSampleTime=-1  VariantActivationTime=update diagram  Latency=0  AutoFrameSizeCalculation=off
      link override defval: Value=KINP_PDUMCUHVLoopSta_enum_defval
      link override ovrdflg: Value=KINP_PDUMCUHVLoopSta_enum_ovrdflg
      link override ovrdval: Value=KINP_PDUMCUHVLoopSta_enum_ovrdval
  PDUMCUPosRlySta : FVT_lib/inp/can_signal_template  SystemSampleTime=-1  VariantActivationTime=update diagram  Latency=0  AutoFrameSizeCalculation=off
      link override defval: Value=KINP_PDUMCUPosRlySta_enum_defval
      link override ovrdflg: Value=KINP_PDUMCUPosRlySta_enum_ovrdflg
      link override ovrdval: Value=KINP_PDUMCUPosRlySta_enum_ovrdval
  PDUMCUPreRlySta : FVT_lib/inp/can_signal_template  SystemSampleTime=-1  VariantActivationTime=update diagram  Latency=0  AutoFrameSizeCalculation=off
      link override defval: Value=KINP_PDUMCUPreRlySta_enum_defval
      link override ovrdflg: Value=KINP_PDUMCUPreRlySta_enum_ovrdflg
      link override ovrdval: Value=KINP_PDUMCUPreRlySta_enum_ovrdval
  PDUSelfChkSta : FVT_lib/inp/can_signal_template  SystemSampleTime=-1  VariantActivationTime=update diagram  Latency=0  AutoFrameSizeCalculation=off
      link override defval: Value=KINP_PDUSelfChkSta_enum_defval
      link override ovrdflg: Value=KINP_PDUSelfChkSta_enum_ovrdflg
      link override ovrdval: Value=KINP_PDUSelfChkSta_enum_ovrdval
  Terminator_{1..20} (20 alike) : Terminator
  True_VHAL_DCDCEnSta_enum : Constant  Value=TRUE  OutDataTypeStr=boolean
  True_VHAL_DCDCErrLvSta_enum : Constant  Value=TRUE  OutDataTypeStr=boolean
  True_VHAL_DCDCOutVolSta_V : Constant  Value=TRUE  OutDataTypeStr=boolean
  True_VHAL_DCDCTempSta_C : Constant  Value=TRUE  OutDataTypeStr=boolean
  True_VHAL_EACEnSta_enum : Constant  Value=TRUE  OutDataTypeStr=boolean
  True_VHAL_EACErrLvSta_enum : Constant  Value=TRUE  OutDataTypeStr=boolean
  True_VHAL_EACInvTempSta_C : Constant  Value=TRUE  OutDataTypeStr=boolean
  True_VHAL_EHPSEnSta_enum : Constant  Value=TRUE  OutDataTypeStr=boolean
  True_VHAL_EHPSErrLvSta_enum : Constant  Value=TRUE  OutDataTypeStr=boolean
  True_VHAL_EHPSInvTempSta_C : Constant  Value=TRUE  OutDataTypeStr=boolean
  True_VHAL_EHPSMotorSpdSta_rpm : Constant  Value=TRUE  OutDataTypeStr=boolean
  True_VHAL_PDUACRlySta_enum : Constant  Value=TRUE  OutDataTypeStr=boolean
  True_VHAL_PDUDCDCEACEHPSHVLoopSta_enum : Constant  Value=TRUE  OutDataTypeStr=boolean
  True_VHAL_PDUDCDCEACEHPSPreRlySta_enum : Constant  Value=TRUE  OutDataTypeStr=boolean
  True_VHAL_PDUDCDCEACEHPSRlySta_enum : Constant  Value=TRUE  OutDataTypeStr=boolean
  True_VHAL_PDUHVILSta_enum : Constant  Value=TRUE  OutDataTypeStr=boolean
  True_VHAL_PDUMCUHVLoopSta_enum : Constant  Value=TRUE  OutDataTypeStr=boolean
  True_VHAL_PDUMCUPosRlySta_enum : Constant  Value=TRUE  OutDataTypeStr=boolean
  True_VHAL_PDUMCUPreRlySta_enum : Constant  Value=TRUE  OutDataTypeStr=boolean
  True_VHAL_PDUSelfChkSta_enum : Constant  Value=TRUE  OutDataTypeStr=boolean
  slr1_{1..20} (20 alike) : BusSelector  OutputSignals=VINP_CANMsgValidzGWCANRr1C500_flg
  slr_VHAL_DCDCEnSta_enum : BusSelector  OutputSignals=VHAL_DCDCEnSta_enum
  slr_VHAL_DCDCErrLvSta_enum : BusSelector  OutputSignals=VHAL_DCDCErrLvSta_enum
  slr_VHAL_DCDCOutVolSta_V : BusSelector  OutputSignals=VHAL_DCDCOutVolSta_V
  slr_VHAL_DCDCTempSta_C : BusSelector  OutputSignals=VHAL_DCDCTempSta_C
  slr_VHAL_EACEnSta_enum : BusSelector  OutputSignals=VHAL_EACEnSta_enum
  slr_VHAL_EACErrLvSta_enum : BusSelector  OutputSignals=VHAL_EACErrLvSta_enum
  slr_VHAL_EACInvTempSta_C : BusSelector  OutputSignals=VHAL_EACInvTempSta_C
  slr_VHAL_EHPSEnSta_enum : BusSelector  OutputSignals=VHAL_EHPSEnSta_enum
  slr_VHAL_EHPSErrLvSta_enum : BusSelector  OutputSignals=VHAL_EHPSErrLvSta_enum
  slr_VHAL_EHPSInvTempSta_C : BusSelector  OutputSignals=VHAL_EHPSInvTempSta_C
  slr_VHAL_EHPSMotorSpdSta_rpm : BusSelector  OutputSignals=VHAL_EHPSMotorSpdSta_rpm
  slr_VHAL_PDUACRlySta_enum : BusSelector  OutputSignals=VHAL_PDUACRlySta_enum
  slr_VHAL_PDUDCDCEACEHPSHVLoopSta_enum : BusSelector  OutputSignals=VHAL_PDUDCDCEACEHPSHVLoopSta_enum
  slr_VHAL_PDUDCDCEACEHPSPreRlySta_enum : BusSelector  OutputSignals=VHAL_PDUDCDCEACEHPSPreRlySta_enum
  slr_VHAL_PDUDCDCEACEHPSRlySta_enum : BusSelector  OutputSignals=VHAL_PDUDCDCEACEHPSRlySta_enum
  slr_VHAL_PDUHVILSta_enum : BusSelector  OutputSignals=VHAL_PDUHVILSta_enum
  slr_VHAL_PDUMCUHVLoopSta_enum : BusSelector  OutputSignals=VHAL_PDUMCUHVLoopSta_enum
  slr_VHAL_PDUMCUPosRlySta_enum : BusSelector  OutputSignals=VHAL_PDUMCUPosRlySta_enum
  slr_VHAL_PDUMCUPreRlySta_enum : BusSelector  OutputSignals=VHAL_PDUMCUPreRlySta_enum
  slr_VHAL_PDUSelfChkSta_enum : BusSelector  OutputSignals=VHAL_PDUSelfChkSta_enum
  VINP_DCDCEnSta_enum : Outport
  VINP_DCDCErrLvSta_enum : Outport  Port=2
  VINP_DCDCOutVolSta_V : Outport  Port=3
  VINP_DCDCTempSta_C : Outport  Port=4
  VINP_EACEnSta_enum : Outport  Port=5
  VINP_EACErrLvSta_enum : Outport  Port=6
  VINP_EACInvTempSta_C : Outport  Port=7
  VINP_EHPSEnSta_enum : Outport  Port=8
  VINP_EHPSErrLvSta_enum : Outport  Port=9
  VINP_EHPSInvTempSta_C : Outport  Port=10
  VINP_EHPSMotorSpdSta_rpm : Outport  Port=11
  VINP_PDUACRlySta_enum : Outport  Port=12
  VINP_PDUDCDCEACEHPSHVLoopSta_enum : Outport  Port=13
  VINP_PDUDCDCEACEHPSPreRlySta_enum : Outport  Port=14
  VINP_PDUDCDCEACEHPSRlySta_enum : Outport  Port=15
  VINP_PDUHVILSta_enum : Outport  Port=16
  VINP_PDUMCUHVLoopSta_enum : Outport  Port=17
  VINP_PDUMCUPosRlySta_enum : Outport  Port=18
  VINP_PDUMCUPreRlySta_enum : Outport  Port=19
  VINP_PDUSelfChkSta_enum : Outport  Port=20
  wires:
  BHAL_outputs/1 -> [BHAL_outputs]
  inp_CanValid_bus/1 -> [inp_CanValid_bus]
  [BHAL_outputs] -> slr_VHAL_DCDCEnSta_enum/1
  slr_VHAL_DCDCEnSta_enum/1 -> DCDCEnSta/1  "<VHAL_DCDCEnSta_enum>"
  True_VHAL_DCDCEnSta_enum/1 -> DCDCEnSta/2
  [inp_CanValid_bus] -> slr1_1/1
  slr1_1/1 -> DCDCEnSta/3  "<VINP_CANMsgValidzGWCANRr1C500_flg>"
  DCDCEnSta/1 -> VINP_DCDCEnSta_enum/1  "VINP_DCDCEnSta_enum"
  DCDCEnSta/2 -> Terminator_1/1
  [BHAL_outputs] -> slr_VHAL_DCDCErrLvSta_enum/1
  slr_VHAL_DCDCErrLvSta_enum/1 -> DCDCErrLvSta/1  "<VHAL_DCDCErrLvSta_enum>"
  True_VHAL_DCDCErrLvSta_enum/1 -> DCDCErrLvSta/2
  [inp_CanValid_bus] -> slr1_2/1
  slr1_2/1 -> DCDCErrLvSta/3  "<VINP_CANMsgValidzGWCANRr1C500_flg>"
  DCDCErrLvSta/1 -> VINP_DCDCErrLvSta_enum/1  "VINP_DCDCErrLvSta_enum"
  DCDCErrLvSta/2 -> Terminator_2/1
  [BHAL_outputs] -> slr_VHAL_DCDCOutVolSta_V/1
  slr_VHAL_DCDCOutVolSta_V/1 -> DCDCOutVolSta/1  "<VHAL_DCDCOutVolSta_V>"
  True_VHAL_DCDCOutVolSta_V/1 -> DCDCOutVolSta/2
  [inp_CanValid_bus] -> slr1_3/1
  slr1_3/1 -> DCDCOutVolSta/3  "<VINP_CANMsgValidzGWCANRr1C500_flg>"
  DCDCOutVolSta/1 -> VINP_DCDCOutVolSta_V/1  "VINP_DCDCOutVolSta_V"
  DCDCOutVolSta/2 -> Terminator_3/1
  [BHAL_outputs] -> slr_VHAL_DCDCTempSta_C/1
  slr_VHAL_DCDCTempSta_C/1 -> DCDCTempSta/1  "<VHAL_DCDCTempSta_C>"
  True_VHAL_DCDCTempSta_C/1 -> DCDCTempSta/2
  [inp_CanValid_bus] -> slr1_4/1
  slr1_4/1 -> DCDCTempSta/3  "<VINP_CANMsgValidzGWCANRr1C500_flg>"
  DCDCTempSta/1 -> VINP_DCDCTempSta_C/1  "VINP_DCDCTempSta_C"
  DCDCTempSta/2 -> Terminator_4/1
  [BHAL_outputs] -> slr_VHAL_EACEnSta_enum/1
  slr_VHAL_EACEnSta_enum/1 -> EACEnSta/1  "<VHAL_EACEnSta_enum>"
  True_VHAL_EACEnSta_enum/1 -> EACEnSta/2
  [inp_CanValid_bus] -> slr1_5/1
  slr1_5/1 -> EACEnSta/3  "<VINP_CANMsgValidzGWCANRr1C500_flg>"
  EACEnSta/1 -> VINP_EACEnSta_enum/1  "VINP_EACEnSta_enum"
  EACEnSta/2 -> Terminator_5/1
  [BHAL_outputs] -> slr_VHAL_EACErrLvSta_enum/1
  slr_VHAL_EACErrLvSta_enum/1 -> EACErrLvSta/1  "<VHAL_EACErrLvSta_enum>"
  True_VHAL_EACErrLvSta_enum/1 -> EACErrLvSta/2
  [inp_CanValid_bus] -> slr1_6/1
  slr1_6/1 -> EACErrLvSta/3  "<VINP_CANMsgValidzGWCANRr1C500_flg>"
  EACErrLvSta/1 -> VINP_EACErrLvSta_enum/1  "VINP_EACErrLvSta_enum"
  EACErrLvSta/2 -> Terminator_6/1
  [BHAL_outputs] -> slr_VHAL_EACInvTempSta_C/1
  slr_VHAL_EACInvTempSta_C/1 -> EACInvTempSta/1  "<VHAL_EACInvTempSta_C>"
  True_VHAL_EACInvTempSta_C/1 -> EACInvTempSta/2
  [inp_CanValid_bus] -> slr1_7/1
  slr1_7/1 -> EACInvTempSta/3  "<VINP_CANMsgValidzGWCANRr1C500_flg>"
  EACInvTempSta/1 -> VINP_EACInvTempSta_C/1  "VINP_EACInvTempSta_C"
  EACInvTempSta/2 -> Terminator_7/1
  [BHAL_outputs] -> slr_VHAL_EHPSEnSta_enum/1
  slr_VHAL_EHPSEnSta_enum/1 -> EHPSEnSta/1  "<VHAL_EHPSEnSta_enum>"
  True_VHAL_EHPSEnSta_enum/1 -> EHPSEnSta/2
  [inp_CanValid_bus] -> slr1_8/1
  slr1_8/1 -> EHPSEnSta/3  "<VINP_CANMsgValidzGWCANRr1C500_flg>"
  EHPSEnSta/1 -> VINP_EHPSEnSta_enum/1  "VINP_EHPSEnSta_enum"
  EHPSEnSta/2 -> Terminator_8/1
  [BHAL_outputs] -> slr_VHAL_EHPSErrLvSta_enum/1
  slr_VHAL_EHPSErrLvSta_enum/1 -> EHPSErrLvSta/1  "<VHAL_EHPSErrLvSta_enum>"
  True_VHAL_EHPSErrLvSta_enum/1 -> EHPSErrLvSta/2
  [inp_CanValid_bus] -> slr1_9/1
  slr1_9/1 -> EHPSErrLvSta/3  "<VINP_CANMsgValidzGWCANRr1C500_flg>"
  EHPSErrLvSta/1 -> VINP_EHPSErrLvSta_enum/1  "VINP_EHPSErrLvSta_enum"
  EHPSErrLvSta/2 -> Terminator_9/1
  [BHAL_outputs] -> slr_VHAL_EHPSInvTempSta_C/1
  slr_VHAL_EHPSInvTempSta_C/1 -> EHPSInvTempSta/1  "<VHAL_EHPSInvTempSta_C>"
  True_VHAL_EHPSInvTempSta_C/1 -> EHPSInvTempSta/2
  [inp_CanValid_bus] -> slr1_10/1
  slr1_10/1 -> EHPSInvTempSta/3  "<VINP_CANMsgValidzGWCANRr1C500_flg>"
  EHPSInvTempSta/1 -> VINP_EHPSInvTempSta_C/1  "VINP_EHPSInvTempSta_C"
  EHPSInvTempSta/2 -> Terminator_10/1
  [BHAL_outputs] -> slr_VHAL_EHPSMotorSpdSta_rpm/1
  slr_VHAL_EHPSMotorSpdSta_rpm/1 -> EHPSMotorSpdSta/1  "<VHAL_EHPSMotorSpdSta_rpm>"
  True_VHAL_EHPSMotorSpdSta_rpm/1 -> EHPSMotorSpdSta/2
  [inp_CanValid_bus] -> slr1_11/1
  slr1_11/1 -> EHPSMotorSpdSta/3  "<VINP_CANMsgValidzGWCANRr1C500_flg>"
  EHPSMotorSpdSta/1 -> VINP_EHPSMotorSpdSta_rpm/1  "VINP_EHPSMotorSpdSta_rpm"
  EHPSMotorSpdSta/2 -> Terminator_11/1
  [BHAL_outputs] -> slr_VHAL_PDUACRlySta_enum/1
  slr_VHAL_PDUACRlySta_enum/1 -> PDUACRlySta/1  "<VHAL_PDUACRlySta_enum>"
  True_VHAL_PDUACRlySta_enum/1 -> PDUACRlySta/2
  [inp_CanValid_bus] -> slr1_12/1
  slr1_12/1 -> PDUACRlySta/3  "<VINP_CANMsgValidzGWCANRr1C500_flg>"
  PDUACRlySta/1 -> VINP_PDUACRlySta_enum/1  "VINP_PDUACRlySta_enum"
  PDUACRlySta/2 -> Terminator_12/1
  [BHAL_outputs] -> slr_VHAL_PDUDCDCEACEHPSHVLoopSta_enum/1
  slr_VHAL_PDUDCDCEACEHPSHVLoopSta_enum/1 -> PDUDCDCEACEHPSHVLoopSta/1  "<VHAL_PDUDCDCEACEHPSHVLoopSta_enum>"
  True_VHAL_PDUDCDCEACEHPSHVLoopSta_enum/1 -> PDUDCDCEACEHPSHVLoopSta/2
  [inp_CanValid_bus] -> slr1_13/1
  slr1_13/1 -> PDUDCDCEACEHPSHVLoopSta/3  "<VINP_CANMsgValidzGWCANRr1C500_flg>"
  PDUDCDCEACEHPSHVLoopSta/1 -> VINP_PDUDCDCEACEHPSHVLoopSta_enum/1  "VINP_PDUDCDCEACEHPSHVLoopSta_enum"
  PDUDCDCEACEHPSHVLoopSta/2 -> Terminator_13/1
  [BHAL_outputs] -> slr_VHAL_PDUDCDCEACEHPSPreRlySta_enum/1
  slr_VHAL_PDUDCDCEACEHPSPreRlySta_enum/1 -> PDUDCDCEACEHPSPreRlySta/1  "<VHAL_PDUDCDCEACEHPSPreRlySta_enum>"
  True_VHAL_PDUDCDCEACEHPSPreRlySta_enum/1 -> PDUDCDCEACEHPSPreRlySta/2
  [inp_CanValid_bus] -> slr1_14/1
  slr1_14/1 -> PDUDCDCEACEHPSPreRlySta/3  "<VINP_CANMsgValidzGWCANRr1C500_flg>"
  PDUDCDCEACEHPSPreRlySta/1 -> VINP_PDUDCDCEACEHPSPreRlySta_enum/1  "VINP_PDUDCDCEACEHPSPreRlySta_enum"
  PDUDCDCEACEHPSPreRlySta/2 -> Terminator_14/1
  [BHAL_outputs] -> slr_VHAL_PDUDCDCEACEHPSRlySta_enum/1
  slr_VHAL_PDUDCDCEACEHPSRlySta_enum/1 -> PDUDCDCEACEHPSRlySta/1  "<VHAL_PDUDCDCEACEHPSRlySta_enum>"
  True_VHAL_PDUDCDCEACEHPSRlySta_enum/1 -> PDUDCDCEACEHPSRlySta/2
  [inp_CanValid_bus] -> slr1_15/1
  slr1_15/1 -> PDUDCDCEACEHPSRlySta/3  "<VINP_CANMsgValidzGWCANRr1C500_flg>"
  PDUDCDCEACEHPSRlySta/1 -> VINP_PDUDCDCEACEHPSRlySta_enum/1  "VINP_PDUDCDCEACEHPSRlySta_enum"
  PDUDCDCEACEHPSRlySta/2 -> Terminator_15/1
  [BHAL_outputs] -> slr_VHAL_PDUHVILSta_enum/1
  slr_VHAL_PDUHVILSta_enum/1 -> PDUHVILSta/1  "<VHAL_PDUHVILSta_enum>"
  True_VHAL_PDUHVILSta_enum/1 -> PDUHVILSta/2
  [inp_CanValid_bus] -> slr1_16/1
  slr1_16/1 -> PDUHVILSta/3  "<VINP_CANMsgValidzGWCANRr1C500_flg>"
  PDUHVILSta/1 -> VINP_PDUHVILSta_enum/1  "VINP_PDUHVILSta_enum"
  PDUHVILSta/2 -> Terminator_16/1
  [BHAL_outputs] -> slr_VHAL_PDUMCUHVLoopSta_enum/1
  slr_VHAL_PDUMCUHVLoopSta_enum/1 -> PDUMCUHVLoopSta/1  "<VHAL_PDUMCUHVLoopSta_enum>"
  True_VHAL_PDUMCUHVLoopSta_enum/1 -> PDUMCUHVLoopSta/2
  [inp_CanValid_bus] -> slr1_17/1
  slr1_17/1 -> PDUMCUHVLoopSta/3  "<VINP_CANMsgValidzGWCANRr1C500_flg>"
  PDUMCUHVLoopSta/1 -> VINP_PDUMCUHVLoopSta_enum/1  "VINP_PDUMCUHVLoopSta_enum"
  PDUMCUHVLoopSta/2 -> Terminator_17/1
  [BHAL_outputs] -> slr_VHAL_PDUMCUPosRlySta_enum/1
  slr_VHAL_PDUMCUPosRlySta_enum/1 -> PDUMCUPosRlySta/1  "<VHAL_PDUMCUPosRlySta_enum>"
  True_VHAL_PDUMCUPosRlySta_enum/1 -> PDUMCUPosRlySta/2
  [inp_CanValid_bus] -> slr1_18/1
  slr1_18/1 -> PDUMCUPosRlySta/3  "<VINP_CANMsgValidzGWCANRr1C500_flg>"
  PDUMCUPosRlySta/1 -> VINP_PDUMCUPosRlySta_enum/1  "VINP_PDUMCUPosRlySta_enum"
  PDUMCUPosRlySta/2 -> Terminator_18/1
  [BHAL_outputs] -> slr_VHAL_PDUMCUPreRlySta_enum/1
  slr_VHAL_PDUMCUPreRlySta_enum/1 -> PDUMCUPreRlySta/1  "<VHAL_PDUMCUPreRlySta_enum>"
  True_VHAL_PDUMCUPreRlySta_enum/1 -> PDUMCUPreRlySta/2
  [inp_CanValid_bus] -> slr1_19/1
  slr1_19/1 -> PDUMCUPreRlySta/3  "<VINP_CANMsgValidzGWCANRr1C500_flg>"
  PDUMCUPreRlySta/1 -> VINP_PDUMCUPreRlySta_enum/1  "VINP_PDUMCUPreRlySta_enum"
  PDUMCUPreRlySta/2 -> Terminator_19/1
  [BHAL_outputs] -> slr_VHAL_PDUSelfChkSta_enum/1
  slr_VHAL_PDUSelfChkSta_enum/1 -> PDUSelfChkSta/1  "<VHAL_PDUSelfChkSta_enum>"
  True_VHAL_PDUSelfChkSta_enum/1 -> PDUSelfChkSta/2
  [inp_CanValid_bus] -> slr1_20/1
  slr1_20/1 -> PDUSelfChkSta/3  "<VINP_CANMsgValidzGWCANRr1C500_flg>"
  PDUSelfChkSta/1 -> VINP_PDUSelfChkSta_enum/1  "VINP_PDUSelfChkSta_enum"
  PDUSelfChkSta/2 -> Terminator_20/1
